simulink model "time_response"  (R2015a)
settings: Solver=ode4  StartTime=0.0  StopTime=5  FixedStep=0.01  RelTol=1e-3
values from neighbouring files (symbols this model uses):
  A = [ ... (first row only)    [ex_expm.m]    (also in ex_residue.m; mimo_test.m; plant.m = [0 1)
  B = [ ... (first row only)    [mimo_test.m]    (also in plant.m = [0 1]')
  C = [ ... (first row only)    [mimo_test.m]    (also in plant.m = [1 0])
  D = [ ... (first row only)    [mimo_test.m]    (also in plant.m = 0)
settings Model: Creator=shohei  LastModifiedBy=shohei

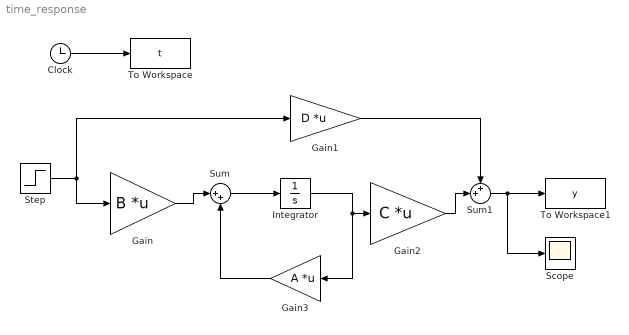
== system time_response ==
  Clock : Clock
  Gain : Gain  Gain=B  Multiplication=Matrix(K*u)
  Gain1 : Gain  Gain=D  Multiplication=Matrix(K*u)
  Gain2 : Gain  Gain=C  Multiplication=Matrix(K*u)
  Gain3 : Gain  Gain=A  Multiplication=Matrix(K*u)
  Integrator : Integrator
  Scope : Scope
  Step : Step  SampleTime=0
  Sum : Sum  Inputs=|++
  Sum1 : Sum  Inputs=++|
  To Workspace : ToWorkspace  VariableName=t  SaveFormat=Timeseries  SampleTime=-1
  To Workspace1 : ToWorkspace  VariableName=y  SaveFormat=Timeseries  SampleTime=-1
  wires:
  Clock/1 -> To Workspace/1
  Step/1 -> Gain/1, Gain1/1
  Gain/1 -> Sum/1
  Sum/1 -> Integrator/1
  Integrator/1 -> Gain2/1, Gain3/1
  Gain3/1 -> Sum/2
  Sum1/1 -> Scope/1, To Workspace1/1
  Gain1/1 -> Sum1/1
  Gain2/1 -> Sum1/2
